simulink model "MapaLogistico"  (R2024b)
settings: Solver=VariableStepAuto  StartTime=0.0  StopTime=10.0  RelTol=1e-3
settings Model: Creator=Miguel  LastModifiedBy=Miguel

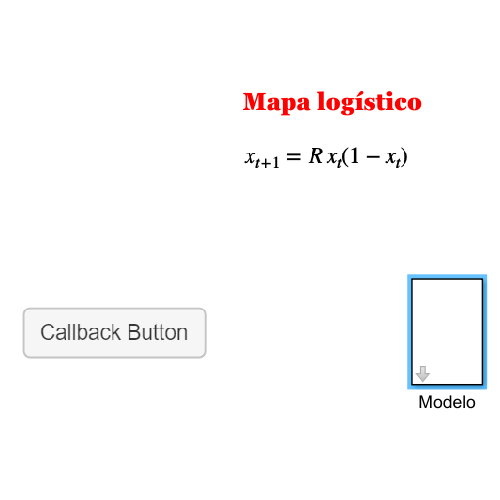
[thumbnail: Simulink's stored preview of the top-level diagram]
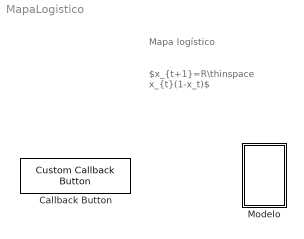
== system MapaLogistico ==
  note: $x_{t+1}=R\thinspace x_{t}(1-x_t)$
  note: Mapa logístico
  Callback Button : CustomCallbackButton  Configuration="{\"components\":[{\"name\":\"BackgroundImageComponent\",\"settings\":{\"image\":{\"size\":[0,0],\"src\":\"default\",\"srcOrientation\":\"Right\"},\"position\":[0,0,1,1]}},{\"name\":\"ButtonStateComponent\",\"settings\":{\"buttonType\":\"momentary\",\"clickFcn\":\"close all\\n\\nx = out.xt;\\nt = 0:length(x)-1;\\n\\nplot(t,x,'b','LineWidth',3)\\ngrid on\\nxlim([0,length(x)-1])\\nylim([0,1])\\nxlabel('$t$','Interpreter','latex','FontSize',14)\\nylabel('$x_{t}$','Interpreter','latex','FontSize',14)\\n\\nx1 = out.xt1;\\nR = out.R;\\n\\n% Curva teórica\\nxt = linspace(0,1,500);\\ny = R*xt.*(1-xt);\\nfigure()\\nplot(xt,y,'b','LineWidth',3)\\nhold \\nxlabel('$x_t$','Interpreter','latex','FontSize',14)\\nylabel('$x_{t+1}$','Interpreter','latex','FontSize',14)\\ntitle('Diagrama de telaraña','Interpreter','latex','FontSize',14)\\nxlim([0,1])\\nylim([0,1])\\n\\nfor k=1:length(x)\\n    plot(x(k),x1(k),'go','MarkerFaceColor','g')\\nend\\n\\ngrid on\\nhold off\",\"onValue\":1,\"position\":[0,0,1,1],\"pressDelay\":\"500\",\"pressFcn\":\"\",\"repeatInterval\":\"0\",\"states\":[{\"horizontalAlignment\":\"center\",\"image\":{\"position\":[0,0,1,1],\"size\":[1,1],\"src\":\"default\",\"srcOrientation\":\"Right\"},\"label\":{\"color\":[0.01176470588,0.01176470588,0.01176470588,1],\"icon\":{\"size\":[0,0],\"src\":\"default\",\"srcOrientation\":\"Right\"},\"iconOffset\":0,\"iconPlacement\":\"left\",\"opacity\":1,\"show\":true,\"text\":{\"content\":\"Callback Button\",\"font\":\"Helvetica\"}},\"labelOffset\":[0,0],\"verticalAlignment\":\"middle\"},{\"horizontalAlignment\":\"center\",\"image\":{\"position\":[0,0,1,1],\"size\":[1,1],\"src\":\"default\",\"srcOrientation\":\"Right\"},\"label\":{\"color\":[0.01176470588,0.01176470588,0.01176470588,1],\"icon\":{\"size\":[0,0],\"src\":\"default\",\"srcOrientation\":\"Right\"},\"iconOffset\":0,\"iconPlacement\":\"left\",\"opacity\":1,\"show\":true,\"text\":{\"content\":\"Callback Button\",\"font\":\"Helvetica\"}},\"labelOffset\":[0,0],\"verticalAlignment\":\"middle\"},{\"horizontalAlignment\":\"center\",\"image\":{\"position\":[0,0,1,1],\"size\":[1,1],\"src\":\"default\",\"srcOrientation\":\"Right\"},\"label\":{\"color\":[0.01176470588,0.01176470588,0.01176470588,1],\"icon\":{\"size\":[0,0],\"src\":\"default\",\"srcOrientation\":\"Right\"},\"iconOffset\":0,\"iconPlacement\":\"left\",\"opacity\":1,\"show\":true,\"text\":{\"content\":\"Callback Button\",\"font\":\"Helvetica\"}},\"labelOffset\":[0,0],\"verticalAlignment\":\"middle\"},{\"horizontalAlignment\":\"center\",\"image\":{\"position\":[0,0,1,1],\"size\":[1,1],\"src\":\"default\",\"srcOrientation\":\"Right\"},\"label\":{\"color\":[0.01176470588,0.01176470588,0.01176470588,1],\"icon\":{\"size\":[0,0],\"src\":\"default\",\"srcOrientation\":\"Right\"},\"iconOffset\":0,\"iconPlacement\":\"left\",\"opacity\":1,\"show\":true,\"text\":{\"content\":\"Callback Button\",\"font\":\"Helvetica\"}},\"labelOffset\":[0,0],\"verticalAlignment\":\"middle\"}]}},{\"name\":\"ForegroundImageComponent\",\"settings\":{\"image\":{\"size\":[0,0],\"src\":\"default\",\"srcOrientation\":\"Right\"},\"isForeground\":1,\"position\":[0,0,1,1]}}],\"settings\":{\"BindingType\":\"standalone\",\"backgroundColor\":[244,244,244,1],\"backgroundOffset\":0.2,\"backgroundOpacity\":1,\"fixedAspectRatio\":\"off\",\"foregroundColor\":[0.01176470588,0.01176470588,0.01176470588,1],\"migratedFromLegacy\":true,\"useBackgroundColor\":true,\"variant\":\"callback\",\"version\":\"R2023a\"},\"type\":\"Button\"}"  CustomBackgroundColor="{\"color\":[0.9568627451,0.9568627451,0.9568627451],\"show\":true}"
  Modelo : Subsystem  mask{R=3.6}

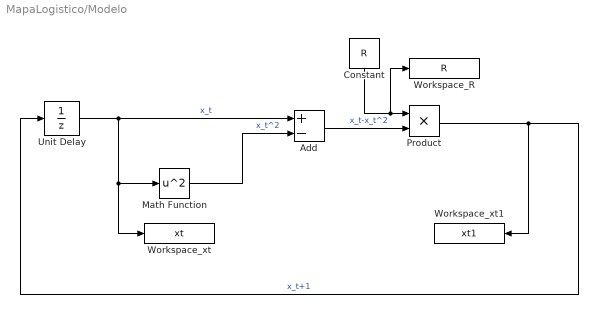
== system MapaLogistico/Modelo ==
  Add : Sum  Inputs=+-
  Constant : Constant  Value=R
  Math Function : Math  Operator=square
  Product : Product
  Unit Delay : UnitDelay  InitialCondition=0.8  SampleTime=-1  HasFrameUpgradeWarning=on
  Workspace_R : ToWorkspace  VariableName=R  SampleTime=-1
  Workspace_xt : ToWorkspace  VariableName=xt  SampleTime=-1
  Workspace_xt1 : ToWorkspace  VariableName=xt1  SampleTime=-1
  wires:
  Unit Delay/1 -> Workspace_xt/1, Math Function/1, Add/1  "x_t"
  Product/1 -> Workspace_xt1/1, Unit Delay/1  "x_t+1"
  Math Function/1 -> Add/2  "x_t^2"
  Constant/1 -> Workspace_R/1, Product/1
  Add/1 -> Product/2  "x_t-x_t^2"
